simulink model "gm_soc_dvbs2_fpga"  (R2025b)
settings: Solver=VariableStepAuto  StartTime=0.0  StopTime=10.0  RelTol=1e-3
InitFcn:
  | soc_dvbs2_init;
undefined symbols (not defined in the file or in its folder): Add, coefficientsLog, coefficientsSqrt1, coefficientsSqrt2, dataBits, Deinterleaver, designMultirateFIR, noisePow, Shift, Short, soc_dvbs2_designFIRFilter, soc_dvbs2_txPacketBits, syncWord, txDataOut, txFiltCoeff, XData
libraries: simulink x304, hdlsllib x265, dspsigops x15, dsphdlfiltering2 x8, hdlmdlgenlib x6, dsphdlsigops2 x5, commseqgen3 x5, dsphdlmathfun2 x3, hwlogicconnlib x2, whdledac x2, commhdlcrc x2, whdlutilities x1
(part 30 of 36)

== system gm_soc_dvbs2_fpga/DVBS2/DVBS2 TxRx/DVB-S2 HDL Receiver/Synchronizer and PL Header Decoder/Time Frequency and Coarse Phase Synchronizer/Time and Coarse Frequency Synchronizer/PL Data Descrambler and Pilot Valid Indicator/Pilot Valid Indicator ==
  note: Hold pilotsEnable signal after endOfPLSC
  note: Hold pilotEnable signal
  pilotEnable : Inport  OutDataTypeStr=boolean  PortDimensions=1  SampleTime=2.5e-07
  validIn : Inport  Port=2  OutDataTypeStr=boolean  PortDimensions=1  SampleTime=2.5e-07
  endOfSOFIn : Inport  Port=3  OutDataTypeStr=boolean  PortDimensions=1  SampleTime=2.5e-07
  endOfPLSC : Inport  Port=4  OutDataTypeStr=boolean  PortDimensions=1  SampleTime=2.5e-07
  Compare To Constant2 : simulink/Logic and Bit Operations/Compare To Constant  relop=>=  const=config.PilotMinIdx  OutDataTypeStr=boolean
  Compare To Constant3 : simulink/Logic and Bit Operations/Compare To Constant  relop=<=  const=config.PilotMaxIdx  OutDataTypeStr=boolean
  Delay{1..4} (4 alike) : Delay  DelayLength=config.SOFLength
  Delay{5..14,19} (11 alike) : Delay  DelayLength=1
  Delay15 : Delay
  Delay16 : Delay
  Delay17 : Delay
  Logical Operator1 : Logic  Inputs=3  AllPortsSameDT=off  OutDataTypeStr=boolean
  Logical Operator2 : Logic  AllPortsSameDT=off  OutDataTypeStr=boolean
  Logical Operator3 : Logic  AllPortsSameDT=off  OutDataTypeStr=boolean
  PilotIdx Counter : hdlsllib/Sources/HDL Counter  CountType=Count limited  CountInit=0  CountStep=1  CountMax=config.PilotMaxIdx  CountFromType=Initial value  CountFrom=0  CountResetPort=on  CountLoadPort=off  CountEnbPort=on  CountDirPort=off  CountHitOutputPort=off  CountDataType=Unsigned  CountWordLen=nextpow2(config.PilotMaxIdx)  CountFracLen=0  CountSampTime=1
  Unit Delay Enabled Resettable Synchronous : hdlsllib/Discrete/Unit Delay Enabled Resettable Synchronous  InitialCondition=0.0  SampleTime=-1
  Unit Delay Enabled Resettable Synchronous1 : hdlsllib/Discrete/Unit Delay Enabled Resettable Synchronous  InitialCondition=0.0  SampleTime=-1
  pilotValid : Outport  SampleTime=2.5e-07
  pilotIdx : Outport  Port=2  SampleTime=2.5e-07
  endOfSOF : Outport  Port=3  SampleTime=2.5e-07
  wires:
  Logical Operator1/1 -> Delay16/1
  Delay10/1 -> Delay15/1
  endOfPLSC/1 -> Delay3/1
  validIn/1 -> Delay4/1
  Compare To Constant3/1 -> Logical Operator3/1
  Compare To Constant2/1 -> Delay11/1
  endOfSOFIn/1 -> Unit Delay Enabled Resettable Synchronous1/3, Delay2/1, Unit Delay Enabled Resettable Synchronous/3
  Delay1/1 -> Unit Delay Enabled Resettable Synchronous/1
  pilotEnable/1 -> Delay1/1
  Delay4/1 -> Delay7/1, PilotIdx Counter/2
  Delay3/1 -> Logical Operator2/1, PilotIdx Counter/1
  Delay2/1 -> Unit Delay Enabled Resettable Synchronous/2, Delay9/1
  Unit Delay Enabled Resettable Synchronous1/1 -> Delay8/1
  PilotIdx Counter/1 -> Delay5/1, Delay19/1, Delay6/1
  Delay7/1 -> Logical Operator3/2
  Delay9/1 -> Delay14/1
  Delay5/1 -> Compare To Constant2/1
  Unit Delay Enabled Resettable Synchronous/1 -> Logical Operator2/2
  Delay19/1 -> Delay10/1
  Delay6/1 -> Compare To Constant3/1
  Delay14/1 -> Delay17/1
  Logical Operator2/1 -> Unit Delay Enabled Resettable Synchronous1/2, Unit Delay Enabled Resettable Synchronous1/1
  Delay17/1 -> endOfSOF/1
  Delay15/1 -> pilotIdx/1
  Logical Operator3/1 -> Delay12/1
  Delay8/1 -> Delay13/1
  Delay11/1 -> Logical Operator1/1
  Delay16/1 -> pilotValid/1
  Delay12/1 -> Logical Operator1/2
  Delay13/1 -> Logical Operator1/3

== system gm_soc_dvbs2_fpga/DVBS2/DVBS2 TxRx/DVB-S2 HDL Receiver/Synchronizer and PL Header Decoder/Time Frequency and Coarse Phase Synchronizer/Time and Coarse Frequency Synchronizer/Symbol Synchronizer/Gardner TED ==
  data : Inport  OutDataTypeStr=fixdt(1, 22, 13)  PortDimensions=1  SampleTime=6.25e-08
      settings: SignalType=complex
  strobe : Inport  Port=2  OutDataTypeStr=boolean  PortDimensions=1  SampleTime=6.25e-08
  Constant : Constant  Value=0  OutDataTypeStr=fixdt(1, 46, 26)  SampleTime=-1
  Delay10 : Delay  DelayLength=4
  GTED : Subsystem
  Switch : Switch  Criteria=u2 ~= 0  OutDataTypeStr=fixdt(1, 46, 26)  InputSameDT=off
  e : Outport  SampleTime=6.25e-08  VectorParamsAs1DForOutWhenUnconnected=off
  wires:
  GTED/1(Out1) -> Switch/1
  data/1 -> GTED/1(In1)
  strobe/1 -> Delay10/1
  Delay10/1 -> Switch/2
  Switch/1 -> e/1
  Constant/1 -> Switch/3

== system gm_soc_dvbs2_fpga/DVBS2/DVBS2 TxRx/DVB-S2 HDL Receiver/Synchronizer and PL Header Decoder/Time Frequency and Coarse Phase Synchronizer/Time and Coarse Frequency Synchronizer/Symbol Synchronizer/Interpolation Control ==
  Delta : Inport  OutDataTypeStr=fixdt(1, 11, 10)  PortDimensions=1  SampleTime=6.25e-08
  Interpolation Control : MATLAB Function
  mu : Outport  SampleTime=6.25e-08
  Underflow : Outport  Port=2  SampleTime=6.25e-08
  wires:
  Interpolation Control/2(Underflow) -> Underflow/1
  Interpolation Control/1(mu) -> mu/1
  Delta/1 -> Interpolation Control/1(Delta)

== system gm_soc_dvbs2_fpga/DVBS2/DVBS2 TxRx/DVB-S2 HDL Receiver/Synchronizer and PL Header Decoder/Time Frequency and Coarse Phase Synchronizer/Time and Coarse Frequency Synchronizer/Symbol Synchronizer/Interpolation Filter ==
  In : Inport  OutDataTypeStr=fixdt(1, 18, 13)  PortDimensions=1  SampleTime=6.25e-08
      settings: SignalType=complex
  mu : Inport  Port=2  OutDataTypeStr=fixdt(1, 11, 10)  PortDimensions=1  SampleTime=6.25e-08
  Delay{,5..9,11..18} (14 alike) : Delay
  Delay{1..4,10} (5 alike) : Delay  DelayLength=1  InitialCondition=0
  Delay{19..36} (18 alike) : Delay  DelayLength=1
  Gain : Gain  Gain=1/2  ParamDataTypeStr=fixdt(0,1,1)  OutDataTypeStr=fixdt(1, 18, 13)
  Product1 : Product  OutDataTypeStr=fixdt(1, 18, 13)  RndMeth=Zero
  Product2 : Product  OutDataTypeStr=fixdt(1, 21, 13)  RndMeth=Zero
  Sum1 : Sum  Inputs=-+|  OutDataTypeStr=fixdt(1, 19, 13)
  Sum10 : Sum  Inputs=|++  OutDataTypeStr=fixdt(1, 20, 13)
  Sum2 : Sum  Inputs=+|+  OutDataTypeStr=fixdt(1, 22, 13)
  Sum3 : Sum  Inputs=+|+  OutDataTypeStr=fixdt(1, 21, 13)
  Sum4 : Sum  Inputs=|+-  OutDataTypeStr=fixdt(1, 21, 13)
  Sum5 : Sum  Inputs=-+|  OutDataTypeStr=fixdt(1, 20, 13)
  Sum6 : Sum  Inputs=+|+  OutDataTypeStr=fixdt(1, 18, 13)  SaturateOnIntegerOverflow=on
  Sum7 : Sum  Inputs=+-|  OutDataTypeStr=fixdt(1, 21, 13)
  Sum9 : Sum  Inputs=+-  OutDataTypeStr=fixdt(1, 19, 13)
  interpolant : Outport  SampleTime=6.25e-08
  wires:
  Delay10/1 -> Delay23/1
  In/1 -> Gain/1, Delay1/1
  Delay1/1 -> Delay36/1
  Product2/1 -> Delay/1
  Sum3/1 -> Delay6/1
  Delay35/1 -> Sum9/2, Delay2/1, Delay30/1
  Sum5/1 -> Delay25/1
  Sum10/1 -> Delay22/1
  Gain/1 -> Delay35/1
  Delay36/1 -> Sum9/1, Delay33/1
  Sum9/1 -> Delay32/1
  Delay19/1 -> Delay24/1
  Delay33/1 -> Delay10/1
  Delay2/1 -> Delay31/1
  Delay18/1 -> Delay12/1
  Delay32/1 -> Sum10/1
  Delay17/1 -> Sum7/1
  Delay31/1 -> Sum1/1, Delay3/1, Sum10/2
  Delay16/1 -> Sum7/2
  Delay30/1 -> Sum1/2
  Delay23/1 -> Delay28/1
  Delay15/1 -> Product1/1
  Delay3/1 -> Delay21/1
  Sum4/1 -> Delay27/1
  Sum1/1 -> Delay20/1
  Delay11/1 -> Sum3/1
  mu/1 -> Delay34/1
  Delay22/1 -> Sum4/1
  Delay28/1 -> Delay18/1
  Delay21/1 -> Sum4/2, Delay4/1, Sum5/1
  Delay20/1 -> Sum5/2
  Delay34/1 -> Delay29/1
  Delay4/1 -> Delay26/1
  Delay29/1 -> Delay19/1
  Delay27/1 -> Delay17/1
  Delay12/1 -> Delay8/1
  Delay26/1 -> Sum6/1, Delay16/1
  Delay25/1 -> Sum6/2
  Delay8/1 -> Delay5/1
  Sum2/1 -> interpolant/1
  Delay6/1 -> Product2/1
  Product1/1 -> Delay9/1
  Sum6/1 -> Delay15/1
  Delay24/1 -> Delay14/1
  Sum7/1 -> Delay11/1
  Delay14/1 -> Product1/2, Delay13/1
  Delay13/1 -> Delay7/1
  Delay9/1 -> Sum3/2
  Delay5/1 -> Sum2/1
  Delay7/1 -> Product2/2
  Delay/1 -> Sum2/2

== system gm_soc_dvbs2_fpga/DVBS2/DVBS2 TxRx/DVB-S2 HDL Receiver/Synchronizer and PL Header Decoder/Time Frequency and Coarse Phase Synchronizer/Time and Coarse Frequency Synchronizer/Symbol Synchronizer/Loop Filter ==
  e : Inport  OutDataTypeStr=fixdt(1, 46, 26)  PortDimensions=1  SampleTime=6.25e-08
  Add : Sum  OutDataTypeStr=fixdt(1, 47, 26)  AccumDataTypeStr=fixdt(1, 47, 26)  SampleTime=6.25e-08
  Add2 : Sum  OutDataTypeStr=fixdt(1, 46, 26)  AccumDataTypeStr=fixdt(1, 47, 26)  SampleTime=6.25e-08
  Data Type Conversion17 : DataTypeConversion  OutDataTypeStr=fixdt(1, 11, 10)  SampleTime=6.25e-08  SaturateOnIntegerOverflow=off  RndMeth=Floor
  Delay{,1,4,6} (4 alike) : Delay  DelayLength=double(1)  InitialCondition=0  SampleTime=6.25e-08
  Delay2 : Delay  DelayLength=double(2)  InitialCondition=0  SampleTime=6.25e-08
  Delay3 : Delay  DelayLength=double(2)  InitialCondition=0  SampleTime=6.25e-08
  Delay5 : Delay  DelayLength=double(2)  InitialCondition=0  SampleTime=6.25e-08
  K1 : Gain  Gain="fi(0,1,24,24,\"hex\",\"fd7e6b\")"  ParamDataTypeStr=fixdt(1, 24, 24)  OutDataTypeStr=fixdt(1, 46, 26)  SampleTime=6.25e-08
  K2 : Gain  Gain="fi(0,1,24,24,\"hex\",\"fff928\")"  ParamDataTypeStr=fixdt(1, 24, 24)  OutDataTypeStr=fixdt(1, 46, 26)  SampleTime=6.25e-08
  v : Outport  SampleTime=6.25e-08
  wires:
  Delay2/1 -> K2/1, K1/1
  e/1 -> Delay2/1
  Data Type Conversion17/1 -> v/1
  Delay5/1 -> Delay6/1
  Delay3/1 -> Delay1/1
  K1/1 -> Delay3/1
  Delay/1 -> Add2/2
  Delay6/1 -> Add2/1
  K2/1 -> Delay5/1
  Delay1/1 -> Add/1
  Add2/1 -> Delay/1, Delay4/1
  Add/1 -> Data Type Conversion17/1
  Delay4/1 -> Add/2

== system gm_soc_dvbs2_fpga/DVBS2/DVBS2 TxRx/DVB-S2 HDL Receiver/Synchronizer and PL Header Decoder/Time Frequency and Coarse Phase Synchronizer/Time and Coarse Frequency Synchronizer/Symbol Synchronizer/Rate Handle ==
  dataIn : Inport  OutDataTypeStr=fixdt(1, 18, 13)  PortDimensions=1  SampleTime=6.25e-08
      settings: SignalType=complex
  strobe : Inport  Port=2  OutDataTypeStr=boolean  PortDimensions=1  SampleTime=6.25e-08
  validIn : Inport  Port=3  OutDataTypeStr=boolean  PortDimensions=1  SampleTime=6.25e-08
  Compare To Constant : simulink/Logic and Bit Operations/Compare To Constant  relop===  const=config.SamplesPerSymbol - 1  OutDataTypeStr=boolean
  Downsample : DownSample  N=config.SamplesPerSymbol  RateOptions=Allow multirate processing
  Downsample1 : DownSample  N=config.SamplesPerSymbol  RateOptions=Allow multirate processing
  FIFO : Subsystem
  HDL Counter : hdlsllib/Sources/HDL Counter  CountType=Count limited  CountInit=0  CountStep=1  CountMax=config.SamplesPerSymbol - 1  CountFromType=Initial value  CountFrom=0  CountResetPort=off  CountLoadPort=off  CountEnbPort=on  CountDirPort=off  CountHitOutputPort=off  CountDataType=Unsigned  CountWordLen=nextpow2(config.SamplesPerSymbol - 1)  CountFracLen=0  CountSampTime=1
  Logical Operator : Logic  AllPortsSameDT=off  OutDataTypeStr=boolean
  Unit Delay Enabled Synchronous : hdlsllib/Discrete/Unit Delay Enabled Synchronous  InitialCondition=0.0  SampleTime=-1
  monostable : Subsystem
  dataOut : Outport  SampleTime=2.5e-07
  validOut : Outport  Port=2  SampleTime=2.5e-07
  wires:
  FIFO/1(out) -> Unit Delay Enabled Synchronous/1
  dataIn/1 -> FIFO/1(data)
  validIn/1 -> HDL Counter/1, Logical Operator/1
  HDL Counter/1 -> Compare To Constant/1
  Compare To Constant/1 -> Logical Operator/2
  FIFO/2(outValid) -> Unit Delay Enabled Synchronous/2, monostable/1(trigger)
  strobe/1 -> FIFO/2(push)
  Logical Operator/1 -> FIFO/3(pop)
  Unit Delay Enabled Synchronous/1 -> Downsample/1
  monostable/1(out) -> Downsample1/1
  Downsample/1 -> dataOut/1
  Downsample1/1 -> validOut/1

== system gm_soc_dvbs2_fpga/DVBS2/DVBS2 TxRx/Channel/AWGN Generator/Unit Variance Gaussian Noise/SqrtImplementation/SqrtEval/FunctionEvaluation/1-D Lookup Table ==
  In1 : Inport
  1-D Lookup Table : Lookup_n-D  NumberOfTableDimensions=1  LookupTableObject=''  BreakpointsForDimension1=[0:64]  BreakpointsForDimension1FirstPoint=10  BreakpointsForDimension2FirstPoint=10  BreakpointsForDimension1Spacing=12  BreakpointsForDimension2Spacing=12  IndexSearchMethod=Evenly spaced points  Table=[coefficientsSqrt1(:,1)' 0]  InterpMethod=Flat  InternalRulePriority=Speed  OutDataTypeStr=fixdt(1,13,12)  RndMeth=Simplest
  1-D Lookup Table_pd1 : Delay  DelayLength=1
  Out1 : Outport
  wires:
  1-D Lookup Table/1 -> 1-D Lookup Table_pd1/1  "c1"
  In1/1 -> 1-D Lookup Table/1
  1-D Lookup Table_pd1/1 -> Out1/1

== system gm_soc_dvbs2_fpga/DVBS2/DVBS2 TxRx/Channel/AWGN Generator/Unit Variance Gaussian Noise/SqrtImplementation/SqrtEval/FunctionEvaluation/1-D Lookup Table1 ==
  In1 : Inport
  1-D Lookup Table1 : Lookup_n-D  NumberOfTableDimensions=1  LookupTableObject=''  BreakpointsForDimension1=0:64  BreakpointsForDimension1FirstPoint=10  BreakpointsForDimension2FirstPoint=10  BreakpointsForDimension1Spacing=12  BreakpointsForDimension2Spacing=12  IndexSearchMethod=Evenly spaced points  Table=[coefficientsSqrt1(:,2)' 0]  InterpMethod=Flat  InternalRulePriority=Speed  OutDataTypeStr=fixdt(1,21,20)  RndMeth=Simplest
  1-D Lookup Table1_pd1 : Delay  DelayLength=1
  Out1 : Outport
  wires:
  1-D Lookup Table1_pd1/1 -> Out1/1
  1-D Lookup Table1/1 -> 1-D Lookup Table1_pd1/1  "c0"
  In1/1 -> 1-D Lookup Table1/1

== system gm_soc_dvbs2_fpga/DVBS2/DVBS2 TxRx/Channel/AWGN Generator/Unit Variance Gaussian Noise/SqrtImplementation/SqrtEval/FunctionEvaluation/1-D Lookup Table2 ==
  In1 : Inport
  1-D Lookup Table2 : Lookup_n-D  NumberOfTableDimensions=1  LookupTableObject=''  BreakpointsForDimension1=0:64  BreakpointsForDimension1FirstPoint=10  BreakpointsForDimension2FirstPoint=10  BreakpointsForDimension1Spacing=12  BreakpointsForDimension2Spacing=12  IndexSearchMethod=Evenly spaced points  Table=[coefficientsSqrt2(:,1)' 0]  InterpMethod=Flat  InternalRulePriority=Speed  OutDataTypeStr=fixdt(1,13,12)  RndMeth=Simplest
  1-D Lookup Table2_pd1 : Delay  DelayLength=1
  Out1 : Outport
  wires:
  1-D Lookup Table2/1 -> 1-D Lookup Table2_pd1/1  "c1"
  In1/1 -> 1-D Lookup Table2/1
  1-D Lookup Table2_pd1/1 -> Out1/1

== system gm_soc_dvbs2_fpga/DVBS2/DVBS2 TxRx/Channel/AWGN Generator/Unit Variance Gaussian Noise/SqrtImplementation/SqrtEval/FunctionEvaluation/1-D Lookup Table3 ==
  In1 : Inport
  1-D Lookup Table3 : Lookup_n-D  NumberOfTableDimensions=1  LookupTableObject=''  BreakpointsForDimension1=0:64  BreakpointsForDimension1FirstPoint=10  BreakpointsForDimension2FirstPoint=10  BreakpointsForDimension1Spacing=12  BreakpointsForDimension2Spacing=12  IndexSearchMethod=Evenly spaced points  Table=[coefficientsSqrt2(:,2)' 0]  InterpMethod=Flat  InternalRulePriority=Speed  OutDataTypeStr=fixdt(1,21,20)  RndMeth=Simplest
  1-D Lookup Table3_pd1 : Delay  DelayLength=1
  Out1 : Outport
  wires:
  1-D Lookup Table3_pd1/1 -> Out1/1
  1-D Lookup Table3/1 -> 1-D Lookup Table3_pd1/1  "c0"
  In1/1 -> 1-D Lookup Table3/1

== system gm_soc_dvbs2_fpga/DVBS2/DVBS2 TxRx/DVB-S2 HDL Receiver/Synchronizer and PL Header Decoder/PL Header Recovery/PL Header Decoder/ML Decoder/Compute Euclidean Distance/Add ==
  In1 : Inport  OutDataTypeStr=fixdt('sfix18_En13')
  In2 : Inport  Port=2  OutDataTypeStr=fixdt('sfix18_En12')
  In3 : Inport  Port=3  OutDataTypeStr=fixdt('ufix1')
  Sum2 : Sum  Inputs=+-  OutDataTypeStr=fixdt(1,20,13)  AccumDataTypeStr=fixdt(1,20,13)
  Sum3 : Sum  OutDataTypeStr=fixdt(1,20,13)  AccumDataTypeStr=fixdt(1,20,13)
  Out1 : Outport
  wires:
  In1/1 -> Sum2/1
  In2/1 -> Sum2/2
  Sum2/1 -> Sum3/1
  In3/1 -> Sum3/2
  Sum3/1 -> Out1/1

== system gm_soc_dvbs2_fpga/DVBS2/DVBS2 TxRx/DVB-S2 HDL Receiver/Synchronizer and PL Header Decoder/PL Header Recovery/PL Header Decoder/ML Decoder/Get Min Index/For Each Subsystem1_instance1 ==
  note: For Each
  valueIn : Inport  OutDataTypeStr=fixdt(1, 25, 15)  PortDimensions=[2]  SampleTime=2.5e-07
  idxIn : Inport  Port=2  OutDataTypeStr=fixdt(0, 6, 0)  PortDimensions=[2]  SampleTime=2.5e-07
  Delay{1..9} (9 alike) : Delay  DelayLength=double(1)  InitialCondition=0  SampleTime=2.5e-07
  Relational Operator : RelationalOperator  Operator=<  OutDataTypeStr=boolean  SampleTime=2.5e-07  InputSameDT=off
  Switch : Switch  Criteria=u2 ~= 0  Threshold="fi(0,0,1,0,\"hex\",\"0\")"  OutDataTypeStr=fixdt(1, 25, 15)  SampleTime=2.5e-07  SaturateOnIntegerOverflow=off  InputSameDT=off
  Switch1 : Switch  Criteria=u2 ~= 0  Threshold="fi(0,0,1,0,\"hex\",\"0\")"  OutDataTypeStr=fixdt(0, 6, 0)  SampleTime=2.5e-07  SaturateOnIntegerOverflow=off  InputSameDT=off
  t : Demux  Outputs=2
  t1 : Demux  Outputs=2
  ValueOut : Outport  SampleTime=2.5e-07
  idxOut : Outport  Port=2  SampleTime=2.5e-07
  wires:
  Delay4/1 -> Switch/1
  Delay8/1 -> ValueOut/1
  valueIn/1 -> Delay3/1
  Delay7/1 -> Switch1/3
  idxIn/1 -> Delay1/1
  Delay3/1 -> t1/1
  Delay1/1 -> t/1
  Switch1/1 -> Delay9/1
  t1/1 -> Relational Operator/1, Delay4/1
  Relational Operator/1 -> Delay2/1
  t1/2 -> Delay5/1, Relational Operator/2
  t/1 -> Delay6/1
  t/2 -> Delay7/1
  Delay5/1 -> Switch/3
  Delay2/1 -> Switch/2, Switch1/2
  Delay6/1 -> Switch1/1
  Switch/1 -> Delay8/1
  Delay9/1 -> idxOut/1

== system gm_soc_dvbs2_fpga/DVBS2/DVBS2 TxRx/DVB-S2 HDL Receiver/Synchronizer and PL Header Decoder/PL Header Recovery/PL Header Decoder/ML Decoder/Get Min Index/For Each Subsystem1_instance10 ==
  note: For Each
  valueIn : Inport  OutDataTypeStr=fixdt(1, 25, 15)  PortDimensions=[2]  SampleTime=2.5e-07
  idxIn : Inport  Port=2  OutDataTypeStr=fixdt(0, 6, 0)  PortDimensions=[2]  SampleTime=2.5e-07
  Delay{1..9} (9 alike) : Delay  DelayLength=double(1)  InitialCondition=0  SampleTime=2.5e-07
  Relational Operator : RelationalOperator  Operator=<  OutDataTypeStr=boolean  SampleTime=2.5e-07  InputSameDT=off
  Switch : Switch  Criteria=u2 ~= 0  Threshold="fi(0,0,1,0,\"hex\",\"0\")"  OutDataTypeStr=fixdt(1, 25, 15)  SampleTime=2.5e-07  SaturateOnIntegerOverflow=off  InputSameDT=off
  Switch1 : Switch  Criteria=u2 ~= 0  Threshold="fi(0,0,1,0,\"hex\",\"0\")"  OutDataTypeStr=fixdt(0, 6, 0)  SampleTime=2.5e-07  SaturateOnIntegerOverflow=off  InputSameDT=off
  t : Demux  Outputs=2
  t1 : Demux  Outputs=2
  ValueOut : Outport  SampleTime=2.5e-07
  idxOut : Outport  Port=2  SampleTime=2.5e-07
  wires:
  Delay8/1 -> ValueOut/1
  valueIn/1 -> Delay3/1
  idxIn/1 -> Delay1/1
  t/1 -> Delay6/1
  Switch1/1 -> Delay9/1
  t1/1 -> Relational Operator/1, Delay4/1
  Delay1/1 -> t/1
  Delay3/1 -> t1/1
  t/2 -> Delay7/1
  Delay4/1 -> Switch/1
  t1/2 -> Relational Operator/2, Delay5/1
  Relational Operator/1 -> Delay2/1
  Delay5/1 -> Switch/3
  Delay6/1 -> Switch1/1
  Delay7/1 -> Switch1/3
  Delay2/1 -> Switch/2, Switch1/2
  Switch/1 -> Delay8/1
  Delay9/1 -> idxOut/1

== system gm_soc_dvbs2_fpga/DVBS2/DVBS2 TxRx/DVB-S2 HDL Receiver/Synchronizer and PL Header Decoder/PL Header Recovery/PL Header Decoder/ML Decoder/Get Min Index/For Each Subsystem1_instance11 ==
  note: For Each
  valueIn : Inport  OutDataTypeStr=fixdt(1, 25, 15)  PortDimensions=[2]  SampleTime=2.5e-07
  idxIn : Inport  Port=2  OutDataTypeStr=fixdt(0, 6, 0)  PortDimensions=[2]  SampleTime=2.5e-07
  Delay{1..9} (9 alike) : Delay  DelayLength=double(1)  InitialCondition=0  SampleTime=2.5e-07
  Relational Operator : RelationalOperator  Operator=<  OutDataTypeStr=boolean  SampleTime=2.5e-07  InputSameDT=off
  Switch : Switch  Criteria=u2 ~= 0  Threshold="fi(0,0,1,0,\"hex\",\"0\")"  OutDataTypeStr=fixdt(1, 25, 15)  SampleTime=2.5e-07  SaturateOnIntegerOverflow=off  InputSameDT=off
  Switch1 : Switch  Criteria=u2 ~= 0  Threshold="fi(0,0,1,0,\"hex\",\"0\")"  OutDataTypeStr=fixdt(0, 6, 0)  SampleTime=2.5e-07  SaturateOnIntegerOverflow=off  InputSameDT=off
  t : Demux  Outputs=2
  t1 : Demux  Outputs=2
  ValueOut : Outport  SampleTime=2.5e-07
  idxOut : Outport  Port=2  SampleTime=2.5e-07
  wires:
  Delay8/1 -> ValueOut/1
  valueIn/1 -> Delay3/1
  Delay1/1 -> t/1
  Switch1/1 -> Delay9/1
  t1/1 -> Relational Operator/1, Delay4/1
  Delay3/1 -> t1/1
  idxIn/1 -> Delay1/1
  t1/2 -> Delay5/1, Relational Operator/2
  Relational Operator/1 -> Delay2/1
  Delay4/1 -> Switch/1
  t/1 -> Delay6/1
  t/2 -> Delay7/1
  Delay5/1 -> Switch/3
  Delay2/1 -> Switch/2, Switch1/2
  Delay6/1 -> Switch1/1
  Delay7/1 -> Switch1/3
  Switch/1 -> Delay8/1
  Delay9/1 -> idxOut/1

== system gm_soc_dvbs2_fpga/DVBS2/DVBS2 TxRx/DVB-S2 HDL Receiver/Synchronizer and PL Header Decoder/PL Header Recovery/PL Header Decoder/ML Decoder/Get Min Index/For Each Subsystem1_instance12 ==
  note: For Each
  valueIn : Inport  OutDataTypeStr=fixdt(1, 25, 15)  PortDimensions=[2]  SampleTime=2.5e-07
  idxIn : Inport  Port=2  OutDataTypeStr=fixdt(0, 6, 0)  PortDimensions=[2]  SampleTime=2.5e-07
  Delay{1..9} (9 alike) : Delay  DelayLength=double(1)  InitialCondition=0  SampleTime=2.5e-07
  Relational Operator : RelationalOperator  Operator=<  OutDataTypeStr=boolean  SampleTime=2.5e-07  InputSameDT=off
  Switch : Switch  Criteria=u2 ~= 0  Threshold="fi(0,0,1,0,\"hex\",\"0\")"  OutDataTypeStr=fixdt(1, 25, 15)  SampleTime=2.5e-07  SaturateOnIntegerOverflow=off  InputSameDT=off
  Switch1 : Switch  Criteria=u2 ~= 0  Threshold="fi(0,0,1,0,\"hex\",\"0\")"  OutDataTypeStr=fixdt(0, 6, 0)  SampleTime=2.5e-07  SaturateOnIntegerOverflow=off  InputSameDT=off
  t : Demux  Outputs=2
  t1 : Demux  Outputs=2
  ValueOut : Outport  SampleTime=2.5e-07
  idxOut : Outport  Port=2  SampleTime=2.5e-07
  wires:
  Delay4/1 -> Switch/1
  Delay8/1 -> ValueOut/1
  valueIn/1 -> Delay3/1
  idxIn/1 -> Delay1/1
  Delay3/1 -> t1/1
  Delay1/1 -> t/1
  Switch1/1 -> Delay9/1
  t1/1 -> Delay4/1, Relational Operator/1
  Relational Operator/1 -> Delay2/1
  t1/2 -> Delay5/1, Relational Operator/2
  t/1 -> Delay6/1
  t/2 -> Delay7/1
  Delay5/1 -> Switch/3
  Delay2/1 -> Switch1/2, Switch/2
  Delay6/1 -> Switch1/1
  Delay7/1 -> Switch1/3
  Switch/1 -> Delay8/1
  Delay9/1 -> idxOut/1

== system gm_soc_dvbs2_fpga/DVBS2/DVBS2 TxRx/DVB-S2 HDL Receiver/Synchronizer and PL Header Decoder/PL Header Recovery/PL Header Decoder/ML Decoder/Get Min Index/For Each Subsystem1_instance13 ==
  note: For Each
  valueIn : Inport  OutDataTypeStr=fixdt(1, 25, 15)  PortDimensions=[2]  SampleTime=2.5e-07
  idxIn : Inport  Port=2  OutDataTypeStr=fixdt(0, 6, 0)  PortDimensions=[2]  SampleTime=2.5e-07
  Delay{1..9} (9 alike) : Delay  DelayLength=double(1)  InitialCondition=0  SampleTime=2.5e-07
  Relational Operator : RelationalOperator  Operator=<  OutDataTypeStr=boolean  SampleTime=2.5e-07  InputSameDT=off
  Switch : Switch  Criteria=u2 ~= 0  Threshold="fi(0,0,1,0,\"hex\",\"0\")"  OutDataTypeStr=fixdt(1, 25, 15)  SampleTime=2.5e-07  SaturateOnIntegerOverflow=off  InputSameDT=off
  Switch1 : Switch  Criteria=u2 ~= 0  Threshold="fi(0,0,1,0,\"hex\",\"0\")"  OutDataTypeStr=fixdt(0, 6, 0)  SampleTime=2.5e-07  SaturateOnIntegerOverflow=off  InputSameDT=off
  t : Demux  Outputs=2
  t1 : Demux  Outputs=2
  ValueOut : Outport  SampleTime=2.5e-07
  idxOut : Outport  Port=2  SampleTime=2.5e-07
  wires:
  Delay8/1 -> ValueOut/1
  valueIn/1 -> Delay3/1
  idxIn/1 -> Delay1/1
  t/1 -> Delay6/1
  Switch1/1 -> Delay9/1
  t1/1 -> Delay4/1, Relational Operator/1
  Delay1/1 -> t/1
  Delay3/1 -> t1/1
  t/2 -> Delay7/1
  Delay4/1 -> Switch/1
  t1/2 -> Relational Operator/2, Delay5/1
  Relational Operator/1 -> Delay2/1
  Delay5/1 -> Switch/3
  Delay6/1 -> Switch1/1
  Delay7/1 -> Switch1/3
  Delay2/1 -> Switch/2, Switch1/2
  Switch/1 -> Delay8/1
  Delay9/1 -> idxOut/1

== system gm_soc_dvbs2_fpga/DVBS2/DVBS2 TxRx/DVB-S2 HDL Receiver/Synchronizer and PL Header Decoder/PL Header Recovery/PL Header Decoder/ML Decoder/Get Min Index/For Each Subsystem1_instance14 ==
  note: For Each
  valueIn : Inport  OutDataTypeStr=fixdt(1, 25, 15)  PortDimensions=[2]  SampleTime=2.5e-07
  idxIn : Inport  Port=2  OutDataTypeStr=fixdt(0, 6, 0)  PortDimensions=[2]  SampleTime=2.5e-07
  Delay{1..9} (9 alike) : Delay  DelayLength=double(1)  InitialCondition=0  SampleTime=2.5e-07
  Relational Operator : RelationalOperator  Operator=<  OutDataTypeStr=boolean  SampleTime=2.5e-07  InputSameDT=off
  Switch : Switch  Criteria=u2 ~= 0  Threshold="fi(0,0,1,0,\"hex\",\"0\")"  OutDataTypeStr=fixdt(1, 25, 15)  SampleTime=2.5e-07  SaturateOnIntegerOverflow=off  InputSameDT=off
  Switch1 : Switch  Criteria=u2 ~= 0  Threshold="fi(0,0,1,0,\"hex\",\"0\")"  OutDataTypeStr=fixdt(0, 6, 0)  SampleTime=2.5e-07  SaturateOnIntegerOverflow=off  InputSameDT=off
  t : Demux  Outputs=2
  t1 : Demux  Outputs=2
  ValueOut : Outport  SampleTime=2.5e-07
  idxOut : Outport  Port=2  SampleTime=2.5e-07
  wires:
  valueIn/1 -> Delay3/1
  idxIn/1 -> Delay1/1
  Delay1/1 -> t/1
  Delay3/1 -> t1/1
  t/1 -> Delay6/1
  t1/1 -> Delay4/1, Relational Operator/1
  t/2 -> Delay7/1
  t1/2 -> Relational Operator/2, Delay5/1
  Relational Operator/1 -> Delay2/1
  Delay5/1 -> Switch/3
  Delay6/1 -> Switch1/1
  Switch1/1 -> Delay9/1
  Delay7/1 -> Switch1/3
  Delay2/1 -> Switch/2, Switch1/2
  Delay4/1 -> Switch/1
  Delay8/1 -> ValueOut/1
  Switch/1 -> Delay8/1
  Delay9/1 -> idxOut/1

== system gm_soc_dvbs2_fpga/DVBS2/DVBS2 TxRx/DVB-S2 HDL Receiver/Synchronizer and PL Header Decoder/PL Header Recovery/PL Header Decoder/ML Decoder/Get Min Index/For Each Subsystem1_instance15 ==
  note: For Each
  valueIn : Inport  OutDataTypeStr=fixdt(1, 25, 15)  PortDimensions=[2]  SampleTime=2.5e-07
  idxIn : Inport  Port=2  OutDataTypeStr=fixdt(0, 6, 0)  PortDimensions=[2]  SampleTime=2.5e-07
  Delay{1..9} (9 alike) : Delay  DelayLength=double(1)  InitialCondition=0  SampleTime=2.5e-07
  Relational Operator : RelationalOperator  Operator=<  OutDataTypeStr=boolean  SampleTime=2.5e-07  InputSameDT=off
  Switch : Switch  Criteria=u2 ~= 0  Threshold="fi(0,0,1,0,\"hex\",\"0\")"  OutDataTypeStr=fixdt(1, 25, 15)  SampleTime=2.5e-07  SaturateOnIntegerOverflow=off  InputSameDT=off
  Switch1 : Switch  Criteria=u2 ~= 0  Threshold="fi(0,0,1,0,\"hex\",\"0\")"  OutDataTypeStr=fixdt(0, 6, 0)  SampleTime=2.5e-07  SaturateOnIntegerOverflow=off  InputSameDT=off
  t : Demux  Outputs=2
  t1 : Demux  Outputs=2
  ValueOut : Outport  SampleTime=2.5e-07
  idxOut : Outport  Port=2  SampleTime=2.5e-07
  wires:
  Delay4/1 -> Switch/1
  Delay8/1 -> ValueOut/1
  valueIn/1 -> Delay3/1
  idxIn/1 -> Delay1/1
  Delay3/1 -> t1/1
  Delay1/1 -> t/1
  Switch1/1 -> Delay9/1
  t1/1 -> Relational Operator/1, Delay4/1
  Relational Operator/1 -> Delay2/1
  t1/2 -> Delay5/1, Relational Operator/2
  t/1 -> Delay6/1
  t/2 -> Delay7/1
  Delay5/1 -> Switch/3
  Delay2/1 -> Switch/2, Switch1/2
  Delay6/1 -> Switch1/1
  Delay7/1 -> Switch1/3
  Switch/1 -> Delay8/1
  Delay9/1 -> idxOut/1

== system gm_soc_dvbs2_fpga/DVBS2/DVBS2 TxRx/DVB-S2 HDL Receiver/Synchronizer and PL Header Decoder/PL Header Recovery/PL Header Decoder/ML Decoder/Get Min Index/For Each Subsystem1_instance16 ==
  note: For Each
  valueIn : Inport  OutDataTypeStr=fixdt(1, 25, 15)  PortDimensions=[2]  SampleTime=2.5e-07
  idxIn : Inport  Port=2  OutDataTypeStr=fixdt(0, 6, 0)  PortDimensions=[2]  SampleTime=2.5e-07
  Delay{1..9} (9 alike) : Delay  DelayLength=double(1)  InitialCondition=0  SampleTime=2.5e-07
  Relational Operator : RelationalOperator  Operator=<  OutDataTypeStr=boolean  SampleTime=2.5e-07  InputSameDT=off
  Switch : Switch  Criteria=u2 ~= 0  Threshold="fi(0,0,1,0,\"hex\",\"0\")"  OutDataTypeStr=fixdt(1, 25, 15)  SampleTime=2.5e-07  SaturateOnIntegerOverflow=off  InputSameDT=off
  Switch1 : Switch  Criteria=u2 ~= 0  Threshold="fi(0,0,1,0,\"hex\",\"0\")"  OutDataTypeStr=fixdt(0, 6, 0)  SampleTime=2.5e-07  SaturateOnIntegerOverflow=off  InputSameDT=off
  t : Demux  Outputs=2
  t1 : Demux  Outputs=2
  ValueOut : Outport  SampleTime=2.5e-07
  idxOut : Outport  Port=2  SampleTime=2.5e-07
  wires:
  Delay8/1 -> ValueOut/1
  valueIn/1 -> Delay3/1
  Delay1/1 -> t/1
  Switch1/1 -> Delay9/1
  t1/1 -> Relational Operator/1, Delay4/1
  Delay3/1 -> t1/1
  idxIn/1 -> Delay1/1
  Relational Operator/1 -> Delay2/1
  t1/2 -> Delay5/1, Relational Operator/2
  Delay4/1 -> Switch/1
  t/1 -> Delay6/1
  t/2 -> Delay7/1
  Delay5/1 -> Switch/3
  Delay2/1 -> Switch/2, Switch1/2
  Delay6/1 -> Switch1/1
  Delay7/1 -> Switch1/3
  Switch/1 -> Delay8/1
  Delay9/1 -> idxOut/1

== system gm_soc_dvbs2_fpga/DVBS2/DVBS2 TxRx/DVB-S2 HDL Receiver/Synchronizer and PL Header Decoder/PL Header Recovery/PL Header Decoder/ML Decoder/Get Min Index/For Each Subsystem1_instance2 ==
  note: For Each
  valueIn : Inport  OutDataTypeStr=fixdt(1, 25, 15)  PortDimensions=[2]  SampleTime=2.5e-07
  idxIn : Inport  Port=2  OutDataTypeStr=fixdt(0, 6, 0)  PortDimensions=[2]  SampleTime=2.5e-07
  Delay{1..9} (9 alike) : Delay  DelayLength=double(1)  InitialCondition=0  SampleTime=2.5e-07
  Relational Operator : RelationalOperator  Operator=<  OutDataTypeStr=boolean  SampleTime=2.5e-07  InputSameDT=off
  Switch : Switch  Criteria=u2 ~= 0  Threshold="fi(0,0,1,0,\"hex\",\"0\")"  OutDataTypeStr=fixdt(1, 25, 15)  SampleTime=2.5e-07  SaturateOnIntegerOverflow=off  InputSameDT=off
  Switch1 : Switch  Criteria=u2 ~= 0  Threshold="fi(0,0,1,0,\"hex\",\"0\")"  OutDataTypeStr=fixdt(0, 6, 0)  SampleTime=2.5e-07  SaturateOnIntegerOverflow=off  InputSameDT=off
  t : Demux  Outputs=2
  t1 : Demux  Outputs=2
  ValueOut : Outport  SampleTime=2.5e-07
  idxOut : Outport  Port=2  SampleTime=2.5e-07
  wires:
  Delay8/1 -> ValueOut/1
  valueIn/1 -> Delay3/1
  Delay1/1 -> t/1
  Switch1/1 -> Delay9/1
  t1/1 -> Relational Operator/1, Delay4/1
  Delay3/1 -> t1/1
  idxIn/1 -> Delay1/1
  Relational Operator/1 -> Delay2/1
  t1/2 -> Delay5/1, Relational Operator/2
  Delay4/1 -> Switch/1
  t/1 -> Delay6/1
  t/2 -> Delay7/1
  Delay5/1 -> Switch/3
  Delay2/1 -> Switch/2, Switch1/2
  Delay6/1 -> Switch1/1
  Delay7/1 -> Switch1/3
  Switch/1 -> Delay8/1
  Delay9/1 -> idxOut/1

== system gm_soc_dvbs2_fpga/DVBS2/DVBS2 TxRx/DVB-S2 HDL Receiver/Synchronizer and PL Header Decoder/PL Header Recovery/PL Header Decoder/ML Decoder/Get Min Index/For Each Subsystem1_instance3 ==
  note: For Each
  valueIn : Inport  OutDataTypeStr=fixdt(1, 25, 15)  PortDimensions=[2]  SampleTime=2.5e-07
  idxIn : Inport  Port=2  OutDataTypeStr=fixdt(0, 6, 0)  PortDimensions=[2]  SampleTime=2.5e-07
  Delay{1..9} (9 alike) : Delay  DelayLength=double(1)  InitialCondition=0  SampleTime=2.5e-07
  Relational Operator : RelationalOperator  Operator=<  OutDataTypeStr=boolean  SampleTime=2.5e-07  InputSameDT=off
  Switch : Switch  Criteria=u2 ~= 0  Threshold="fi(0,0,1,0,\"hex\",\"0\")"  OutDataTypeStr=fixdt(1, 25, 15)  SampleTime=2.5e-07  SaturateOnIntegerOverflow=off  InputSameDT=off
  Switch1 : Switch  Criteria=u2 ~= 0  Threshold="fi(0,0,1,0,\"hex\",\"0\")"  OutDataTypeStr=fixdt(0, 6, 0)  SampleTime=2.5e-07  SaturateOnIntegerOverflow=off  InputSameDT=off
  t : Demux  Outputs=2
  t1 : Demux  Outputs=2
  ValueOut : Outport  SampleTime=2.5e-07
  idxOut : Outport  Port=2  SampleTime=2.5e-07
  wires:
  valueIn/1 -> Delay3/1
  idxIn/1 -> Delay1/1
  Delay9/1 -> idxOut/1
  Delay1/1 -> t/1
  Delay3/1 -> t1/1
  t/1 -> Delay6/1
  t1/1 -> Delay4/1, Relational Operator/1
  t/2 -> Delay7/1
  t1/2 -> Relational Operator/2, Delay5/1
  Relational Operator/1 -> Delay2/1
  Delay5/1 -> Switch/3
  Delay6/1 -> Switch1/1
  Switch1/1 -> Delay9/1
  Delay7/1 -> Switch1/3
  Delay2/1 -> Switch/2, Switch1/2
  Delay4/1 -> Switch/1
  Delay8/1 -> ValueOut/1
  Switch/1 -> Delay8/1

== system gm_soc_dvbs2_fpga/DVBS2/DVBS2 TxRx/DVB-S2 HDL Receiver/Synchronizer and PL Header Decoder/PL Header Recovery/PL Header Decoder/ML Decoder/Get Min Index/For Each Subsystem1_instance4 ==
  note: For Each
  valueIn : Inport  OutDataTypeStr=fixdt(1, 25, 15)  PortDimensions=[2]  SampleTime=2.5e-07
  idxIn : Inport  Port=2  OutDataTypeStr=fixdt(0, 6, 0)  PortDimensions=[2]  SampleTime=2.5e-07
  Delay{1..9} (9 alike) : Delay  DelayLength=double(1)  InitialCondition=0  SampleTime=2.5e-07
  Relational Operator : RelationalOperator  Operator=<  OutDataTypeStr=boolean  SampleTime=2.5e-07  InputSameDT=off
  Switch : Switch  Criteria=u2 ~= 0  Threshold="fi(0,0,1,0,\"hex\",\"0\")"  OutDataTypeStr=fixdt(1, 25, 15)  SampleTime=2.5e-07  SaturateOnIntegerOverflow=off  InputSameDT=off
  Switch1 : Switch  Criteria=u2 ~= 0  Threshold="fi(0,0,1,0,\"hex\",\"0\")"  OutDataTypeStr=fixdt(0, 6, 0)  SampleTime=2.5e-07  SaturateOnIntegerOverflow=off  InputSameDT=off
  t : Demux  Outputs=2
  t1 : Demux  Outputs=2
  ValueOut : Outport  SampleTime=2.5e-07
  idxOut : Outport  Port=2  SampleTime=2.5e-07
  wires:
  Delay4/1 -> Switch/1
  Delay8/1 -> ValueOut/1
  valueIn/1 -> Delay3/1
  Delay1/1 -> t/1
  Switch1/1 -> Delay9/1
  t1/1 -> Relational Operator/1, Delay4/1
  Delay3/1 -> t1/1
  idxIn/1 -> Delay1/1
  Relational Operator/1 -> Delay2/1
  t1/2 -> Delay5/1, Relational Operator/2
  t/1 -> Delay6/1
  t/2 -> Delay7/1
  Delay5/1 -> Switch/3
  Delay2/1 -> Switch/2, Switch1/2
  Delay6/1 -> Switch1/1
  Delay7/1 -> Switch1/3
  Switch/1 -> Delay8/1
  Delay9/1 -> idxOut/1

== system gm_soc_dvbs2_fpga/DVBS2/DVBS2 TxRx/DVB-S2 HDL Receiver/Synchronizer and PL Header Decoder/PL Header Recovery/PL Header Decoder/ML Decoder/Get Min Index/For Each Subsystem1_instance5 ==
  note: For Each
  valueIn : Inport  OutDataTypeStr=fixdt(1, 25, 15)  PortDimensions=[2]  SampleTime=2.5e-07
  idxIn : Inport  Port=2  OutDataTypeStr=fixdt(0, 6, 0)  PortDimensions=[2]  SampleTime=2.5e-07
  Delay{1..9} (9 alike) : Delay  DelayLength=double(1)  InitialCondition=0  SampleTime=2.5e-07
  Relational Operator : RelationalOperator  Operator=<  OutDataTypeStr=boolean  SampleTime=2.5e-07  InputSameDT=off
  Switch : Switch  Criteria=u2 ~= 0  Threshold="fi(0,0,1,0,\"hex\",\"0\")"  OutDataTypeStr=fixdt(1, 25, 15)  SampleTime=2.5e-07  SaturateOnIntegerOverflow=off  InputSameDT=off
  Switch1 : Switch  Criteria=u2 ~= 0  Threshold="fi(0,0,1,0,\"hex\",\"0\")"  OutDataTypeStr=fixdt(0, 6, 0)  SampleTime=2.5e-07  SaturateOnIntegerOverflow=off  InputSameDT=off
  t : Demux  Outputs=2
  t1 : Demux  Outputs=2
  ValueOut : Outport  SampleTime=2.5e-07
  idxOut : Outport  Port=2  SampleTime=2.5e-07
  wires:
  Delay8/1 -> ValueOut/1
  valueIn/1 -> Delay3/1
  idxIn/1 -> Delay1/1
  t/1 -> Delay6/1
  Switch1/1 -> Delay9/1
  t1/1 -> Delay4/1, Relational Operator/1
  Delay1/1 -> t/1
  Delay3/1 -> t1/1
  t/2 -> Delay7/1
  Delay4/1 -> Switch/1
  t1/2 -> Relational Operator/2, Delay5/1
  Relational Operator/1 -> Delay2/1
  Delay5/1 -> Switch/3
  Delay6/1 -> Switch1/1
  Delay7/1 -> Switch1/3
  Delay2/1 -> Switch/2, Switch1/2
  Switch/1 -> Delay8/1
  Delay9/1 -> idxOut/1

== system gm_soc_dvbs2_fpga/DVBS2/DVBS2 TxRx/DVB-S2 HDL Receiver/Synchronizer and PL Header Decoder/PL Header Recovery/PL Header Decoder/ML Decoder/Get Min Index/For Each Subsystem1_instance6 ==
  note: For Each
  valueIn : Inport  OutDataTypeStr=fixdt(1, 25, 15)  PortDimensions=[2]  SampleTime=2.5e-07
  idxIn : Inport  Port=2  OutDataTypeStr=fixdt(0, 6, 0)  PortDimensions=[2]  SampleTime=2.5e-07
  Delay{1..9} (9 alike) : Delay  DelayLength=double(1)  InitialCondition=0  SampleTime=2.5e-07
  Relational Operator : RelationalOperator  Operator=<  OutDataTypeStr=boolean  SampleTime=2.5e-07  InputSameDT=off
  Switch : Switch  Criteria=u2 ~= 0  Threshold="fi(0,0,1,0,\"hex\",\"0\")"  OutDataTypeStr=fixdt(1, 25, 15)  SampleTime=2.5e-07  SaturateOnIntegerOverflow=off  InputSameDT=off
  Switch1 : Switch  Criteria=u2 ~= 0  Threshold="fi(0,0,1,0,\"hex\",\"0\")"  OutDataTypeStr=fixdt(0, 6, 0)  SampleTime=2.5e-07  SaturateOnIntegerOverflow=off  InputSameDT=off
  t : Demux  Outputs=2
  t1 : Demux  Outputs=2
  ValueOut : Outport  SampleTime=2.5e-07
  idxOut : Outport  Port=2  SampleTime=2.5e-07
  wires:
  valueIn/1 -> Delay3/1
  Delay9/1 -> idxOut/1
  Delay1/1 -> t/1
  Delay3/1 -> t1/1
  idxIn/1 -> Delay1/1
  t1/1 -> Relational Operator/1, Delay4/1
  Relational Operator/1 -> Delay2/1
  t1/2 -> Delay5/1, Relational Operator/2
  Delay4/1 -> Switch/1
  t/1 -> Delay6/1
  t/2 -> Delay7/1
  Delay5/1 -> Switch/3
  Delay2/1 -> Switch/2, Switch1/2
  Delay6/1 -> Switch1/1
  Switch1/1 -> Delay9/1
  Delay7/1 -> Switch1/3
  Switch/1 -> Delay8/1
  Delay8/1 -> ValueOut/1

== system gm_soc_dvbs2_fpga/DVBS2/DVBS2 TxRx/DVB-S2 HDL Receiver/Synchronizer and PL Header Decoder/PL Header Recovery/PL Header Decoder/ML Decoder/Get Min Index/For Each Subsystem1_instance7 ==
  note: For Each
  valueIn : Inport  OutDataTypeStr=fixdt(1, 25, 15)  PortDimensions=[2]  SampleTime=2.5e-07
  idxIn : Inport  Port=2  OutDataTypeStr=fixdt(0, 6, 0)  PortDimensions=[2]  SampleTime=2.5e-07
  Delay{1..9} (9 alike) : Delay  DelayLength=double(1)  InitialCondition=0  SampleTime=2.5e-07
  Relational Operator : RelationalOperator  Operator=<  OutDataTypeStr=boolean  SampleTime=2.5e-07  InputSameDT=off
  Switch : Switch  Criteria=u2 ~= 0  Threshold="fi(0,0,1,0,\"hex\",\"0\")"  OutDataTypeStr=fixdt(1, 25, 15)  SampleTime=2.5e-07  SaturateOnIntegerOverflow=off  InputSameDT=off
  Switch1 : Switch  Criteria=u2 ~= 0  Threshold="fi(0,0,1,0,\"hex\",\"0\")"  OutDataTypeStr=fixdt(0, 6, 0)  SampleTime=2.5e-07  SaturateOnIntegerOverflow=off  InputSameDT=off
  t : Demux  Outputs=2
  t1 : Demux  Outputs=2
  ValueOut : Outport  SampleTime=2.5e-07
  idxOut : Outport  Port=2  SampleTime=2.5e-07
  wires:
  Delay8/1 -> ValueOut/1
  valueIn/1 -> Delay3/1
  Delay1/1 -> t/1
  Switch1/1 -> Delay9/1
  t1/1 -> Relational Operator/1, Delay4/1
  Delay3/1 -> t1/1
  idxIn/1 -> Delay1/1
  Relational Operator/1 -> Delay2/1
  t1/2 -> Delay5/1, Relational Operator/2
  Delay4/1 -> Switch/1
  t/1 -> Delay6/1
  t/2 -> Delay7/1
  Delay5/1 -> Switch/3
  Delay2/1 -> Switch/2, Switch1/2
  Delay6/1 -> Switch1/1
  Delay7/1 -> Switch1/3
  Switch/1 -> Delay8/1
  Delay9/1 -> idxOut/1

== system gm_soc_dvbs2_fpga/DVBS2/DVBS2 TxRx/DVB-S2 HDL Receiver/Synchronizer and PL Header Decoder/PL Header Recovery/PL Header Decoder/ML Decoder/Get Min Index/For Each Subsystem1_instance8 ==
  note: For Each
  valueIn : Inport  OutDataTypeStr=fixdt(1, 25, 15)  PortDimensions=[2]  SampleTime=2.5e-07
  idxIn : Inport  Port=2  OutDataTypeStr=fixdt(0, 6, 0)  PortDimensions=[2]  SampleTime=2.5e-07
  Delay{1..9} (9 alike) : Delay  DelayLength=double(1)  InitialCondition=0  SampleTime=2.5e-07
  Relational Operator : RelationalOperator  Operator=<  OutDataTypeStr=boolean  SampleTime=2.5e-07  InputSameDT=off
  Switch : Switch  Criteria=u2 ~= 0  Threshold="fi(0,0,1,0,\"hex\",\"0\")"  OutDataTypeStr=fixdt(1, 25, 15)  SampleTime=2.5e-07  SaturateOnIntegerOverflow=off  InputSameDT=off
  Switch1 : Switch  Criteria=u2 ~= 0  Threshold="fi(0,0,1,0,\"hex\",\"0\")"  OutDataTypeStr=fixdt(0, 6, 0)  SampleTime=2.5e-07  SaturateOnIntegerOverflow=off  InputSameDT=off
  t : Demux  Outputs=2
  t1 : Demux  Outputs=2
  ValueOut : Outport  SampleTime=2.5e-07
  idxOut : Outport  Port=2  SampleTime=2.5e-07
  wires:
  Delay8/1 -> ValueOut/1
  valueIn/1 -> Delay3/1
  Delay1/1 -> t/1
  Switch1/1 -> Delay9/1
  t1/1 -> Delay4/1, Relational Operator/1
  Delay3/1 -> t1/1
  idxIn/1 -> Delay1/1
  Relational Operator/1 -> Delay2/1
  t1/2 -> Delay5/1, Relational Operator/2
  Delay4/1 -> Switch/1
  t/1 -> Delay6/1
  t/2 -> Delay7/1
  Delay5/1 -> Switch/3
  Delay2/1 -> Switch/2, Switch1/2
  Delay6/1 -> Switch1/1
  Delay7/1 -> Switch1/3
  Switch/1 -> Delay8/1
  Delay9/1 -> idxOut/1

== system gm_soc_dvbs2_fpga/DVBS2/DVBS2 TxRx/DVB-S2 HDL Receiver/Synchronizer and PL Header Decoder/PL Header Recovery/PL Header Decoder/ML Decoder/Get Min Index/For Each Subsystem1_instance9 ==
  note: For Each
  valueIn : Inport  OutDataTypeStr=fixdt(1, 25, 15)  PortDimensions=[2]  SampleTime=2.5e-07
  idxIn : Inport  Port=2  OutDataTypeStr=fixdt(0, 6, 0)  PortDimensions=[2]  SampleTime=2.5e-07
  Delay{1..9} (9 alike) : Delay  DelayLength=double(1)  InitialCondition=0  SampleTime=2.5e-07
  Relational Operator : RelationalOperator  Operator=<  OutDataTypeStr=boolean  SampleTime=2.5e-07  InputSameDT=off
  Switch : Switch  Criteria=u2 ~= 0  Threshold="fi(0,0,1,0,\"hex\",\"0\")"  OutDataTypeStr=fixdt(1, 25, 15)  SampleTime=2.5e-07  SaturateOnIntegerOverflow=off  InputSameDT=off
  Switch1 : Switch  Criteria=u2 ~= 0  Threshold="fi(0,0,1,0,\"hex\",\"0\")"  OutDataTypeStr=fixdt(0, 6, 0)  SampleTime=2.5e-07  SaturateOnIntegerOverflow=off  InputSameDT=off
  t : Demux  Outputs=2
  t1 : Demux  Outputs=2
  ValueOut : Outport  SampleTime=2.5e-07
  idxOut : Outport  Port=2  SampleTime=2.5e-07
  wires:
  valueIn/1 -> Delay3/1
  Delay9/1 -> idxOut/1
  Delay1/1 -> t/1
  idxIn/1 -> Delay1/1
  Delay3/1 -> t1/1
  Switch1/1 -> Delay9/1
  t1/1 -> Relational Operator/1, Delay4/1
  Relational Operator/1 -> Delay2/1
  t1/2 -> Delay5/1, Relational Operator/2
  Delay4/1 -> Switch/1
  t/1 -> Delay6/1
  t/2 -> Delay7/1
  Delay5/1 -> Switch/3
  Delay2/1 -> Switch/2, Switch1/2
  Delay6/1 -> Switch1/1
  Delay7/1 -> Switch1/3
  Switch/1 -> Delay8/1
  Delay8/1 -> ValueOut/1

== system gm_soc_dvbs2_fpga/DVBS2/DVBS2 TxRx/DVB-S2 HDL Receiver/Synchronizer and PL Header Decoder/PL Header Recovery/PL Header Decoder/ML Decoder/Get Min Index/For Each Subsystem2_instance1 ==
  note: For Each
  valueIn : Inport  OutDataTypeStr=fixdt(1, 25, 15)  PortDimensions=[2]  SampleTime=2.5e-07
  idxIn : Inport  Port=2  OutDataTypeStr=fixdt(0, 6, 0)  PortDimensions=[2]  SampleTime=2.5e-07
  Delay{1..9} (9 alike) : Delay  DelayLength=double(1)  InitialCondition=0  SampleTime=2.5e-07
  Relational Operator : RelationalOperator  Operator=<  OutDataTypeStr=boolean  SampleTime=2.5e-07  InputSameDT=off
  Switch : Switch  Criteria=u2 ~= 0  Threshold="fi(0,0,1,0,\"hex\",\"0\")"  OutDataTypeStr=fixdt(1, 25, 15)  SampleTime=2.5e-07  SaturateOnIntegerOverflow=off  InputSameDT=off
  Switch1 : Switch  Criteria=u2 ~= 0  Threshold="fi(0,0,1,0,\"hex\",\"0\")"  OutDataTypeStr=fixdt(0, 6, 0)  SampleTime=2.5e-07  SaturateOnIntegerOverflow=off  InputSameDT=off
  t : Demux  Outputs=2
  t1 : Demux  Outputs=2
  ValueOut : Outport  SampleTime=2.5e-07
  idxOut : Outport  Port=2  SampleTime=2.5e-07
  wires:
  Delay8/1 -> ValueOut/1
  valueIn/1 -> Delay3/1
  Delay1/1 -> t/1
  Delay3/1 -> t1/1
  Delay7/1 -> Switch1/3
  idxIn/1 -> Delay1/1
  t/1 -> Delay6/1
  Switch1/1 -> Delay9/1
  t1/1 -> Delay4/1, Relational Operator/1
  t/2 -> Delay7/1
  t1/2 -> Relational Operator/2, Delay5/1
  Relational Operator/1 -> Delay2/1
  Delay5/1 -> Switch/3
  Delay6/1 -> Switch1/1
  Delay2/1 -> Switch/2, Switch1/2
  Delay4/1 -> Switch/1
  Switch/1 -> Delay8/1
  Delay9/1 -> idxOut/1

== system gm_soc_dvbs2_fpga/DVBS2/DVBS2 TxRx/DVB-S2 HDL Receiver/Synchronizer and PL Header Decoder/PL Header Recovery/PL Header Decoder/ML Decoder/Get Min Index/For Each Subsystem2_instance2 ==
  note: For Each
  valueIn : Inport  OutDataTypeStr=fixdt(1, 25, 15)  PortDimensions=[2]  SampleTime=2.5e-07
  idxIn : Inport  Port=2  OutDataTypeStr=fixdt(0, 6, 0)  PortDimensions=[2]  SampleTime=2.5e-07
  Delay{1..9} (9 alike) : Delay  DelayLength=double(1)  InitialCondition=0  SampleTime=2.5e-07
  Relational Operator : RelationalOperator  Operator=<  OutDataTypeStr=boolean  SampleTime=2.5e-07  InputSameDT=off
  Switch : Switch  Criteria=u2 ~= 0  Threshold="fi(0,0,1,0,\"hex\",\"0\")"  OutDataTypeStr=fixdt(1, 25, 15)  SampleTime=2.5e-07  SaturateOnIntegerOverflow=off  InputSameDT=off
  Switch1 : Switch  Criteria=u2 ~= 0  Threshold="fi(0,0,1,0,\"hex\",\"0\")"  OutDataTypeStr=fixdt(0, 6, 0)  SampleTime=2.5e-07  SaturateOnIntegerOverflow=off  InputSameDT=off
  t : Demux  Outputs=2
  t1 : Demux  Outputs=2
  ValueOut : Outport  SampleTime=2.5e-07
  idxOut : Outport  Port=2  SampleTime=2.5e-07
  wires:
  Delay8/1 -> ValueOut/1
  valueIn/1 -> Delay3/1
  idxIn/1 -> Delay1/1
  t/1 -> Delay6/1
  Switch1/1 -> Delay9/1
  t1/1 -> Delay4/1, Relational Operator/1
  Delay1/1 -> t/1
  Delay3/1 -> t1/1
  t/2 -> Delay7/1
  Delay4/1 -> Switch/1
  t1/2 -> Relational Operator/2, Delay5/1
  Relational Operator/1 -> Delay2/1
  Delay5/1 -> Switch/3
  Delay6/1 -> Switch1/1
  Delay7/1 -> Switch1/3
  Delay2/1 -> Switch/2, Switch1/2
  Switch/1 -> Delay8/1
  Delay9/1 -> idxOut/1

== system gm_soc_dvbs2_fpga/DVBS2/DVBS2 TxRx/DVB-S2 HDL Receiver/Synchronizer and PL Header Decoder/PL Header Recovery/PL Header Decoder/ML Decoder/Get Min Index/For Each Subsystem2_instance3 ==
  note: For Each
  valueIn : Inport  OutDataTypeStr=fixdt(1, 25, 15)  PortDimensions=[2]  SampleTime=2.5e-07
  idxIn : Inport  Port=2  OutDataTypeStr=fixdt(0, 6, 0)  PortDimensions=[2]  SampleTime=2.5e-07
  Delay{1..9} (9 alike) : Delay  DelayLength=double(1)  InitialCondition=0  SampleTime=2.5e-07
  Relational Operator : RelationalOperator  Operator=<  OutDataTypeStr=boolean  SampleTime=2.5e-07  InputSameDT=off
  Switch : Switch  Criteria=u2 ~= 0  Threshold="fi(0,0,1,0,\"hex\",\"0\")"  OutDataTypeStr=fixdt(1, 25, 15)  SampleTime=2.5e-07  SaturateOnIntegerOverflow=off  InputSameDT=off
  Switch1 : Switch  Criteria=u2 ~= 0  Threshold="fi(0,0,1,0,\"hex\",\"0\")"  OutDataTypeStr=fixdt(0, 6, 0)  SampleTime=2.5e-07  SaturateOnIntegerOverflow=off  InputSameDT=off
  t : Demux  Outputs=2
  t1 : Demux  Outputs=2
  ValueOut : Outport  SampleTime=2.5e-07
  idxOut : Outport  Port=2  SampleTime=2.5e-07
  wires:
  Delay8/1 -> ValueOut/1
  valueIn/1 -> Delay3/1
  Delay1/1 -> t/1
  Delay3/1 -> t1/1
  idxIn/1 -> Delay1/1
  t1/1 -> Relational Operator/1, Delay4/1
  t1/2 -> Delay5/1, Relational Operator/2
  Relational Operator/1 -> Delay2/1
  Delay4/1 -> Switch/1
  t/1 -> Delay6/1
  t/2 -> Delay7/1
  Delay5/1 -> Switch/3
  Delay2/1 -> Switch/2, Switch1/2
  Delay6/1 -> Switch1/1
  Switch1/1 -> Delay9/1
  Delay7/1 -> Switch1/3
  Switch/1 -> Delay8/1
  Delay9/1 -> idxOut/1

== system gm_soc_dvbs2_fpga/DVBS2/DVBS2 TxRx/DVB-S2 HDL Receiver/Synchronizer and PL Header Decoder/PL Header Recovery/PL Header Decoder/ML Decoder/Get Min Index/For Each Subsystem2_instance4 ==
  note: For Each
  valueIn : Inport  OutDataTypeStr=fixdt(1, 25, 15)  PortDimensions=[2]  SampleTime=2.5e-07
  idxIn : Inport  Port=2  OutDataTypeStr=fixdt(0, 6, 0)  PortDimensions=[2]  SampleTime=2.5e-07
  Delay{1..9} (9 alike) : Delay  DelayLength=double(1)  InitialCondition=0  SampleTime=2.5e-07
  Relational Operator : RelationalOperator  Operator=<  OutDataTypeStr=boolean  SampleTime=2.5e-07  InputSameDT=off
  Switch : Switch  Criteria=u2 ~= 0  Threshold="fi(0,0,1,0,\"hex\",\"0\")"  OutDataTypeStr=fixdt(1, 25, 15)  SampleTime=2.5e-07  SaturateOnIntegerOverflow=off  InputSameDT=off
  Switch1 : Switch  Criteria=u2 ~= 0  Threshold="fi(0,0,1,0,\"hex\",\"0\")"  OutDataTypeStr=fixdt(0, 6, 0)  SampleTime=2.5e-07  SaturateOnIntegerOverflow=off  InputSameDT=off
  t : Demux  Outputs=2
  t1 : Demux  Outputs=2
  ValueOut : Outport  SampleTime=2.5e-07
  idxOut : Outport  Port=2  SampleTime=2.5e-07
  wires:
  Delay4/1 -> Switch/1
  Delay8/1 -> ValueOut/1
  valueIn/1 -> Delay3/1
  idxIn/1 -> Delay1/1
  Delay3/1 -> t1/1
  Delay1/1 -> t/1
  Switch1/1 -> Delay9/1
  t1/1 -> Relational Operator/1, Delay4/1
  Relational Operator/1 -> Delay2/1
  t1/2 -> Delay5/1, Relational Operator/2
  t/1 -> Delay6/1
  t/2 -> Delay7/1
  Delay5/1 -> Switch/3
  Delay2/1 -> Switch/2, Switch1/2
  Delay6/1 -> Switch1/1
  Delay7/1 -> Switch1/3
  Switch/1 -> Delay8/1
  Delay9/1 -> idxOut/1

== system gm_soc_dvbs2_fpga/DVBS2/DVBS2 TxRx/DVB-S2 HDL Receiver/Synchronizer and PL Header Decoder/PL Header Recovery/PL Header Decoder/ML Decoder/Get Min Index/For Each Subsystem2_instance5 ==
  note: For Each
  valueIn : Inport  OutDataTypeStr=fixdt(1, 25, 15)  PortDimensions=[2]  SampleTime=2.5e-07
  idxIn : Inport  Port=2  OutDataTypeStr=fixdt(0, 6, 0)  PortDimensions=[2]  SampleTime=2.5e-07
  Delay{1..9} (9 alike) : Delay  DelayLength=double(1)  InitialCondition=0  SampleTime=2.5e-07
  Relational Operator : RelationalOperator  Operator=<  OutDataTypeStr=boolean  SampleTime=2.5e-07  InputSameDT=off
  Switch : Switch  Criteria=u2 ~= 0  Threshold="fi(0,0,1,0,\"hex\",\"0\")"  OutDataTypeStr=fixdt(1, 25, 15)  SampleTime=2.5e-07  SaturateOnIntegerOverflow=off  InputSameDT=off
  Switch1 : Switch  Criteria=u2 ~= 0  Threshold="fi(0,0,1,0,\"hex\",\"0\")"  OutDataTypeStr=fixdt(0, 6, 0)  SampleTime=2.5e-07  SaturateOnIntegerOverflow=off  InputSameDT=off
  t : Demux  Outputs=2
  t1 : Demux  Outputs=2
  ValueOut : Outport  SampleTime=2.5e-07
  idxOut : Outport  Port=2  SampleTime=2.5e-07
  wires:
  Delay8/1 -> ValueOut/1
  valueIn/1 -> Delay3/1
  idxIn/1 -> Delay1/1
  t/1 -> Delay6/1
  Switch1/1 -> Delay9/1
  t1/1 -> Delay4/1, Relational Operator/1
  Delay1/1 -> t/1
  Delay3/1 -> t1/1
  t/2 -> Delay7/1
  Delay4/1 -> Switch/1
  t1/2 -> Relational Operator/2, Delay5/1
  Relational Operator/1 -> Delay2/1
  Delay5/1 -> Switch/3
  Delay6/1 -> Switch1/1
  Delay7/1 -> Switch1/3
  Delay2/1 -> Switch/2, Switch1/2
  Switch/1 -> Delay8/1
  Delay9/1 -> idxOut/1
